simulink model "liq_ofc"  (R2020a)
settings: Solver=VariableStepAuto  StartTime=0.0  StopTime=simulation.stopTime  RelTol=1e-3
values from neighbouring files (symbols this model uses):
  MaxCrossings = 3    [liquid_ofc_detection.m]
  Threshold = 0.1    [liquid_ofc_detection.m]
  tp = 1/2/pi    (= 0.159154943092)    [liquid_ofc_detection.m]
undefined symbols (not defined in the file or in its folder): simulation
libraries: dspsigops x1
settings Model: Creator=FawadFarooq  LastModifiedBy=FawaD KhaN
settings DebuggingCC: SFMachineParentedDataDiag=error

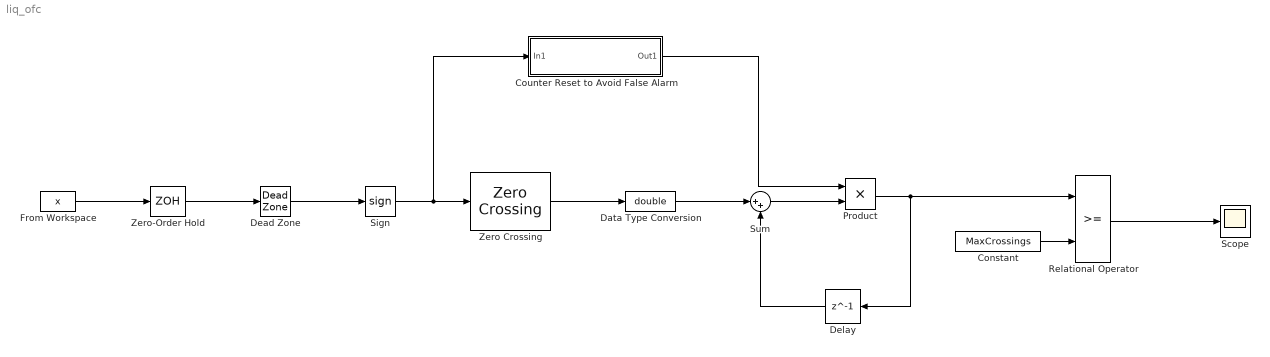
== system liq_ofc ==
  Constant : Constant  Value=MaxCrossings
  Counter Reset to Avoid False Alarm : Subsystem
  Data Type Conversion : DataTypeConversion  OutDataTypeStr=double
  Dead Zone : DeadZone  LowerValue=-Threshold  UpperValue=Threshold  SaturateOnIntegerOverflow=on
  Delay : Delay  DelayLength=1  SampleTime=1/simulation.Fs
  From Workspace : FromWorkspace  VariableName=x  SampleTime=1/simulation.Fs
  Product : Product
  Relational Operator : RelationalOperator  OutDataTypeStr=boolean  RndMeth=Simplest
  Scope : Scope
  Sign : Signum
  Sum : Sum  Inputs=|++
  Zero Crossing : dspsigops/Zero Crossing  InputProcessing=Columns as channels (frame based)
      settings: SourceProductBaseCode=DS
  Zero-Order Hold : ZeroOrderHold  SampleTime=1/simulation.Fs
  wires:
  From Workspace/1 -> Zero-Order Hold/1
  Dead Zone/1 -> Sign/1
  Sign/1 -> Counter Reset to Avoid False Alarm/1(In1), Zero Crossing/1
  Zero Crossing/1 -> Data Type Conversion/1
  Data Type Conversion/1 -> Sum/1
  Zero-Order Hold/1 -> Dead Zone/1
  Delay/1 -> Sum/2
  Sum/1 -> Product/2
  Product/1 -> Delay/1, Relational Operator/1
  Constant/1 -> Relational Operator/2
  Relational Operator/1 -> Scope/1
  Counter Reset to Avoid False Alarm/1(Out1) -> Product/1

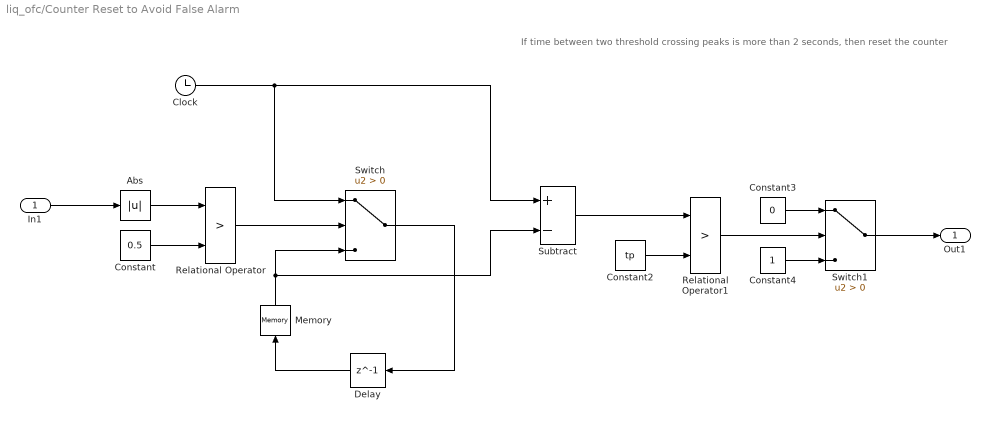
== system liq_ofc/Counter Reset to Avoid False Alarm ==
  note: If time between two threshold crossing peaks is more than 2 seconds, then reset the counter
  In1 : Inport
  Abs : Abs
  Clock : Clock
  Constant : Constant  Value=0.5
  Constant2 : Constant  Value=tp
  Constant3 : Constant  Value=0
  Constant4 : Constant
  Delay : Delay  DelayLength=1  SampleTime=1/simulation.Fs
  Memory : Memory
  Relational Operator : RelationalOperator  Operator=>  OutDataTypeStr=boolean  RndMeth=Simplest
  Relational Operator1 : RelationalOperator  Operator=>  OutDataTypeStr=boolean  RndMeth=Simplest
  Subtract : Sum  Inputs=+-
  Switch : Switch  Criteria=u2 > Threshold
  Switch1 : Switch  Criteria=u2 > Threshold
  Out1 : Outport
  wires:
  Switch1/1 -> Out1/1
  In1/1 -> Abs/1
  Abs/1 -> Relational Operator/1
  Constant/1 -> Relational Operator/2
  Relational Operator/1 -> Switch/2
  Switch/1 -> Delay/1
  Delay/1 -> Memory/1
  Memory/1 -> Subtract/2, Switch/3
  Clock/1 -> Subtract/1, Switch/1
  Subtract/1 -> Relational Operator1/1
  Constant2/1 -> Relational Operator1/2
  Relational Operator1/1 -> Switch1/2
  Constant3/1 -> Switch1/1
  Constant4/1 -> Switch1/3
